simulink model "obieg_pierwotny_add_pressurizer"  (R2016a)
settings: Solver=VariableStepAuto  StartTime=0.0  StopTime=14400  RelTol=1e-3
values from neighbouring files (symbols this model uses):
  c_p_PC = 5415    [unit_1.m]
  c_p_PR = 6873.1    [unit_1.m]
  c_phi_1 = 2.98    [unit_1.m]
  c_phi_2 = -0.008448    [unit_1.m]
  c_psi = 13.75 * (10 ^ 6)    (= 13750000)    [unit_1.m]
  K_T_SG = 9.5296*(10^6)    (= 9529600)    [unit_1.m]
  m_in = 1.4222    [unit_1.m]
  m_out = 2.9722    [unit_1.m]
  N = 99.3    [Unit_3.m]    (also in unit_1.m = 100.3; unit_4.m = 100.8)
  T_PC = 293.03    [unit_1.m]
  T_PC_HL = 293.08    [unit_1.m]
  T_PC_I = 246.1    [unit_1.m]
  T_SG = 255.13    [unit_1.m]
  V0_PC = 242    [unit_1.m]
  W_heat_PR = 1    [unit_1.m]
  W_loss_PC = 2.2469 * (10 ^ 8)    (= 224690000)    [unit_1.m]
  W_loss_PR = 1.6823 * 10^5    (= 168230)    [unit_1.m]
libraries: simulink x2
settings Model: Creator=Michal Chruscinski  LastModifiedBy=Użytkownik
settings GRTTargetCC: GeneratePreprocessorConditionals=Use local settings

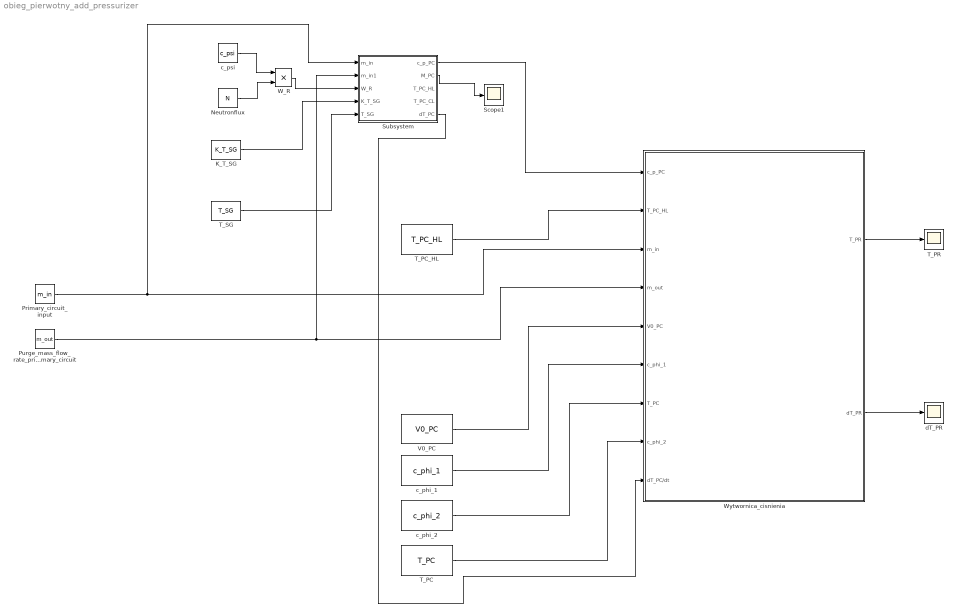
== system obieg_pierwotny_add_pressurizer ==
  K_T_SG : Constant  Value=K_T_SG
  Neutronflux : Constant  Value=N
  Primary_circuit_input : Constant  Value=m_in
  "Purge_mass_flow_rate_primary_circuit " : Constant  Value=m_out
  Scope1 : Scope
  Subsystem : Subsystem
  T_PC : Constant  Value=T_PC
  T_PC_HL : Constant  Value=T_PC_HL
  T_PR : Scope
  T_SG : Constant  Value=T_SG
  V0_PC : Constant  Value=V0_PC
  W_R : Product
  Wytwornica_cisnienia : Subsystem
  c_phi_1 : Constant  Value=c_phi_1
  c_phi_2 : Constant  Value=c_phi_2
  c_psi : Constant  Value=c_psi
  dT_PR : Scope
  wires:
  c_psi/1 -> W_R/1
  Neutronflux/1 -> W_R/2
  W_R/1 -> Subsystem/3(W_R)
  K_T_SG/1 -> Subsystem/4(K_T_SG)
  T_SG/1 -> Subsystem/5(T_SG)
  Subsystem/2(M_PC) -> Scope1/1
  Subsystem/1(c_p_PC) -> Wytwornica_cisnienia/1(c_p_PC)
  c_phi_2/1 -> Wytwornica_cisnienia/7(T_PC)
  T_PC/1 -> Wytwornica_cisnienia/8(c_phi_2)
  T_PC_HL/1 -> Wytwornica_cisnienia/2(T_PC_HL)
  Primary_circuit_input/1 -> Subsystem/1(m_in), Wytwornica_cisnienia/3(m_in)
  "Purge_mass_flow_rate_primary_circuit "/1 -> Wytwornica_cisnienia/4(m_out), Subsystem/2(m_in1)
  V0_PC/1 -> Wytwornica_cisnienia/5(V0_PC)
  c_phi_1/1 -> Wytwornica_cisnienia/6(c_phi_1)
  Wytwornica_cisnienia/1(T_PR) -> T_PR/1
  Wytwornica_cisnienia/2(dT_PR) -> dT_PR/1
  Subsystem/5(dT_PC) -> Wytwornica_cisnienia/9(dT_PC/dt)

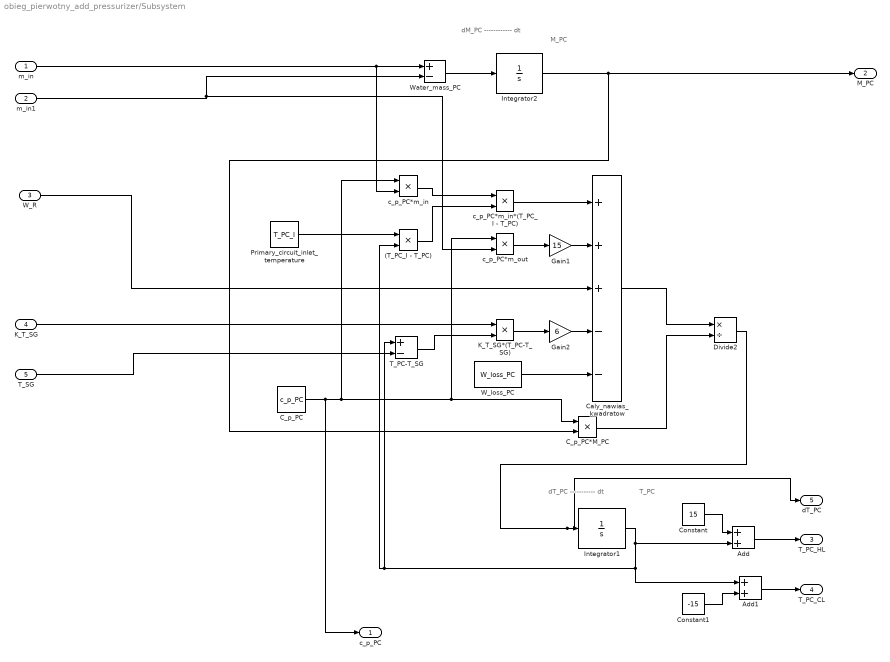
== system obieg_pierwotny_add_pressurizer/Subsystem ==
  note: dM_PC
      | ------------
      |      dt
  note: M_PC
  note: dT_PC
      | -----------
      |     dt
  note: T_PC
  m_in : Inport
  m_in1 : Inport  Port=2
  W_R : Inport  Port=3
  K_T_SG : Inport  Port=4
  T_SG : Inport  Port=5
  (T_PC_I - T_PC) : Product
  Add : Sum
  Add1 : Sum
  C_p_PC : Constant  Value=c_p_PC
  C_p_PC*M_PC : Product
  Caly_nawias_kwadratow : Sum  Inputs=+++--
  Constant : Constant  Value=15
  Constant1 : Constant  Value=-15
  Divide2 : Product  Inputs=*/
  Gain1 : Gain  Gain=15
  Gain2 : Gain  Gain=6
  Integrator1 : Integrator  InitialCondition=278.03
  Integrator2 : Integrator  InitialCondition=200000
  K_T_SG*(T_PC-T_SG) : Product
  Primary_circuit_inlet_temperature : Constant  Value=T_PC_I
  T_PC-T_SG : Sum  Inputs=+-
  W_loss_PC : Constant  Value=W_loss_PC
  Water_mass_PC : Sum  Inputs=+-
  c_p_PC*m_in : Product
  c_p_PC*m_in*(T_PC_I - T_PC) : Product
  c_p_PC*m_out : Product
  c_p_PC : Outport
  M_PC : Outport  Port=2
  T_PC_HL : Outport  Port=3
  T_PC_CL : Outport  Port=4
  dT_PC : Outport  Port=5
  wires:
  m_in/1 -> c_p_PC*m_in/2, Water_mass_PC/1
  Water_mass_PC/1 -> Integrator2/1
  Integrator2/1 -> C_p_PC*M_PC/2, M_PC/1
  C_p_PC/1 -> c_p_PC/1, C_p_PC*M_PC/1, c_p_PC*m_out/1, c_p_PC*m_in/1
  C_p_PC*M_PC/1 -> Divide2/2
  Divide2/1 -> dT_PC/1, Integrator1/1
  Caly_nawias_kwadratow/1 -> Divide2/1
  c_p_PC*m_in*(T_PC_I - T_PC)/1 -> Caly_nawias_kwadratow/1
  c_p_PC*m_in/1 -> c_p_PC*m_in*(T_PC_I - T_PC)/1
  (T_PC_I - T_PC)/1 -> c_p_PC*m_in*(T_PC_I - T_PC)/2
  Primary_circuit_inlet_temperature/1 -> (T_PC_I - T_PC)/1
  c_p_PC*m_out/1 -> Gain1/1
  Gain1/1 -> Caly_nawias_kwadratow/2
  Gain2/1 -> Caly_nawias_kwadratow/4
  K_T_SG*(T_PC-T_SG)/1 -> Gain2/1
  T_PC-T_SG/1 -> K_T_SG*(T_PC-T_SG)/2
  K_T_SG/1 -> K_T_SG*(T_PC-T_SG)/1
  T_SG/1 -> T_PC-T_SG/2
  W_loss_PC/1 -> Caly_nawias_kwadratow/5
  W_R/1 -> Caly_nawias_kwadratow/3
  Constant/1 -> Add/1
  Constant1/1 -> Add1/2
  Integrator1/1 -> Add1/1, (T_PC_I - T_PC)/2, T_PC-T_SG/1, Add/2
  Add1/1 -> T_PC_CL/1
  Add/1 -> T_PC_HL/1
  m_in1/1 -> c_p_PC*m_out/2, Water_mass_PC/2

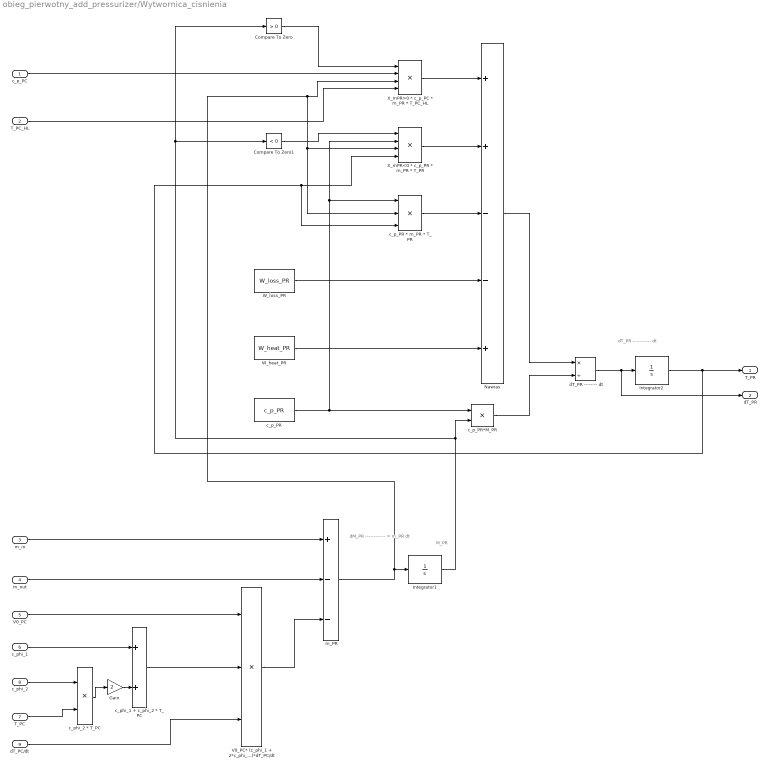
== system obieg_pierwotny_add_pressurizer/Wytwornica_cisnienia ==
  note: dT_PR
      | -----------
      | dt
  note: dM_PR
      | ------------ = m_PR
      |     dt
  note: M_PR
  c_p_PC : Inport
  T_PC_HL : Inport  Port=2
  m_in : Inport  Port=3
  m_out : Inport  Port=4
  V0_PC : Inport  Port=5
  c_phi_1 : Inport  Port=6
  T_PC : Inport  Port=7
  c_phi_2 : Inport  Port=8
  dT_PC/dt : Inport  Port=9
  Compare To Zero : simulink/Logic and Bit Operations/Compare To Zero  relop=>  OutDataTypeStr=boolean
  Compare To Zero1 : simulink/Logic and Bit Operations/Compare To Zero  relop=<  OutDataTypeStr=boolean
  Gain : Gain  Gain=2
  Integrator1 : Integrator  InitialCondition=19400
  Integrator2 : Integrator  InitialCondition=326.57
  Nawias : Sum  Inputs=++--+
  V0_PC* (c_phi_1 + 2*c_phi_2*T_PC)*dT_PC/dt : Product  Inputs=3
  W_heat_PR : Constant  Value=W_heat_PR
  W_loss_PR : Constant  Value=W_loss_PR
  X_mPR<0 * c_p_PR * m_PR * T_PR : Product  Inputs=4
  X_mPR>0 * c_p_PC * m_PR * T_PC_HL : Product  Inputs=4
  c_p_PR : Constant  Value=c_p_PR
  c_p_PR * m_PR * T_PR : Product  Inputs=3
  c_p_PR*M_PR : Product
  "c_phi_1 + c_phi_2 * T_PC " : Sum
  c_phi_2 * T_PC : Product
  dT_PR -------- dt : Product  Inputs=*/
  m_PR : Sum  Inputs=+--
  T_PR : Outport
  dT_PR : Outport  Port=2
  wires:
  c_p_PR*M_PR/1 -> dT_PR -------- dt/2
  Nawias/1 -> dT_PR -------- dt/1
  Integrator1/1 -> Compare To Zero1/1, Compare To Zero/1, c_p_PR*M_PR/2
  c_p_PR/1 -> X_mPR<0 * c_p_PR * m_PR * T_PR/2, c_p_PR * m_PR * T_PR/1, c_p_PR*M_PR/1
  Compare To Zero/1 -> X_mPR>0 * c_p_PC * m_PR * T_PC_HL/1
  X_mPR>0 * c_p_PC * m_PR * T_PC_HL/1 -> Nawias/1
  c_p_PC/1 -> X_mPR>0 * c_p_PC * m_PR * T_PC_HL/2
  m_PR/1 -> X_mPR>0 * c_p_PC * m_PR * T_PC_HL/3, c_p_PR * m_PR * T_PR/2, X_mPR<0 * c_p_PR * m_PR * T_PR/3, Integrator1/1
  T_PC_HL/1 -> X_mPR>0 * c_p_PC * m_PR * T_PC_HL/4
  X_mPR<0 * c_p_PR * m_PR * T_PR/1 -> Nawias/2
  Compare To Zero1/1 -> X_mPR<0 * c_p_PR * m_PR * T_PR/1
  Integrator2/1 -> X_mPR<0 * c_p_PR * m_PR * T_PR/4, c_p_PR * m_PR * T_PR/3, T_PR/1
  c_p_PR * m_PR * T_PR/1 -> Nawias/3
  W_heat_PR/1 -> Nawias/5
  W_loss_PR/1 -> Nawias/4
  m_in/1 -> m_PR/1
  m_out/1 -> m_PR/2
  V0_PC* (c_phi_1 + 2*c_phi_2*T_PC)*dT_PC/dt/1 -> m_PR/3
  V0_PC/1 -> V0_PC* (c_phi_1 + 2*c_phi_2*T_PC)*dT_PC/dt/1
  "c_phi_1 + c_phi_2 * T_PC "/1 -> V0_PC* (c_phi_1 + 2*c_phi_2*T_PC)*dT_PC/dt/2
  c_phi_1/1 -> "c_phi_1 + c_phi_2 * T_PC "/1
  c_phi_2 * T_PC/1 -> Gain/1
  Gain/1 -> "c_phi_1 + c_phi_2 * T_PC "/2
  c_phi_2/1 -> c_phi_2 * T_PC/1
  T_PC/1 -> c_phi_2 * T_PC/2
  dT_PR -------- dt/1 -> dT_PR/1, Integrator2/1
  dT_PC/dt/1 -> V0_PC* (c_phi_1 + 2*c_phi_2*T_PC)*dT_PC/dt/3
